simulink model "Differentialpulsecodemodulation"  (R2021b)
settings: Solver=VariableStepAuto  StartTime=0.0  StopTime=10.0  RelTol=1e-3
libraries: dspquant2 x2, dsparch4 x1, dspsigops x1
settings Model: Creator=hp  LastModifiedBy=hp

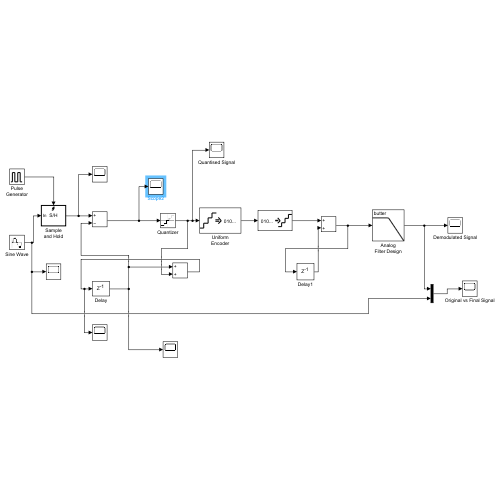
[thumbnail: Simulink's stored preview of the top-level diagram]
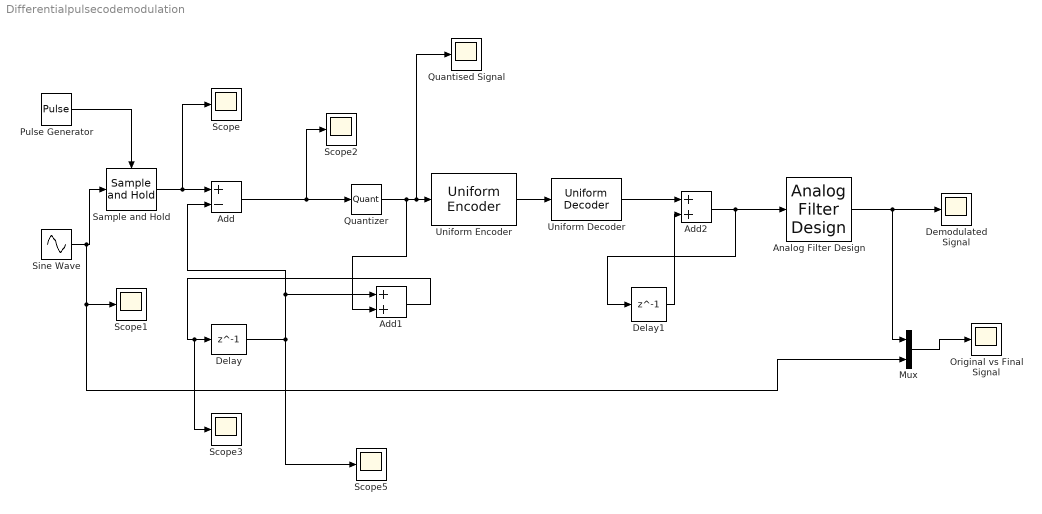
== system Differentialpulsecodemodulation ==
  Add : Sum  Inputs=+-
  Add1 : Sum
  Add2 : Sum
  Analog Filter Design : dsparch4/Analog Filter Design  method=Butterworth  filttype=Lowpass  N=16  Wlo=2*pi*40  Whi=80  Rp=2  Rs=40
  Delay : Delay  DelayLength=1
  Delay1 : Delay  DelayLength=1
  Demodulated Signal : Scope
  Mux : Mux  Inputs=2
  Original vs Final Signal : Scope
  Pulse Generator : DiscretePulseGenerator  PulseType=Time based  Period=1/400  PulseWidth=5
  Quantised Signal : Scope
  Quantizer : Quantizer  QuantizationInterval=0.1
  Sample and Hold : dspsigops/Sample and Hold  trig=Rising edge  initCond=0  latchinput=off
  Scope{,1..3,5} (5 alike) : Scope
  Sine Wave : Sin  Amplitude=3  Frequency=2*pi*2  SampleTime=1/50000
  Uniform Decoder : dspquant2/Uniform Decoder  peak=3  bits=16  overflowMode=Saturate  otype=Double
      settings: SourceProductBaseCode=DS
  Uniform Encoder : dspquant2/Uniform Encoder  peak=3  bits=16  otype=Unsigned integer
  wires:
  Sine Wave/1 -> Mux/2, Scope1/1, Sample and Hold/1
  Pulse Generator/1 -> Sample and Hold/Trigger
  Sample and Hold/1 -> Scope/1, Add/1
  Add/1 -> Scope2/1, Quantizer/1
  Quantizer/1 -> Add1/2, Quantised Signal/1, Uniform Encoder/1
  Delay/1 -> Add1/1, Add/2, Scope5/1
  Add1/1 -> Scope3/1, Delay/1
  Uniform Encoder/1 -> Uniform Decoder/1
  Uniform Decoder/1 -> Add2/1
  Add2/1 -> Analog Filter Design/1, Delay1/1
  Delay1/1 -> Add2/2
  Analog Filter Design/1 -> Mux/1, Demodulated Signal/1
  Mux/1 -> Original vs Final Signal/1
